simulink model "lead"  (Simulink 7.4)
settings: Solver=ode45  StartTime=0.0  StopTime=10.0  RelTol=1e-3
settings Model: Creator=Administrator  LastModifiedBy=Administrator

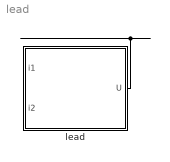
== system lead ==
  lead : Subsystem
  wires:
  ? -> lead/2(i2)
  lead/1(U) -> ?

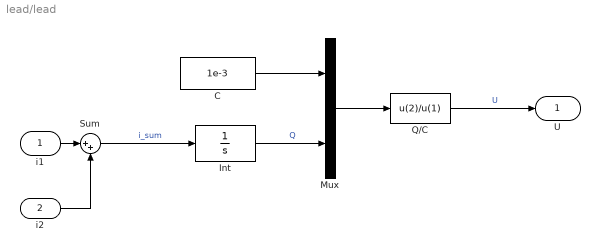
== system lead/lead ==
  i1 : Inport
  i2 : Inport  Port=2
  C : Constant  Value=1e-3  OutDataType=fixdt(1, 16)  OutScaling=2^0
  Int : Integrator
  Mux : Mux  Inputs=2
  Q/C : Fcn  Expr=u(2)/u(1)
  Sum : Sum  Inputs=|++  OutDataType=fixdt(1, 16)  OutScaling=2^0
  U : Outport
  wires:
  Sum/1 -> Int/1  "i_sum"
  Mux/1 -> Q/C/1
  C/1 -> Mux/1
  Int/1 -> Mux/2  "Q"
  Q/C/1 -> U/1  "U"
  i1/1 -> Sum/1
  i2/1 -> Sum/2
